simulink model "SIP_DynSys_Model_V1_0"  (R2024a)
settings: Solver=VariableStepAuto  StartTime=0.0  StopTime=10.0  RelTol=1e-3
settings Model: Creator=yunus  LastModifiedBy=yunus

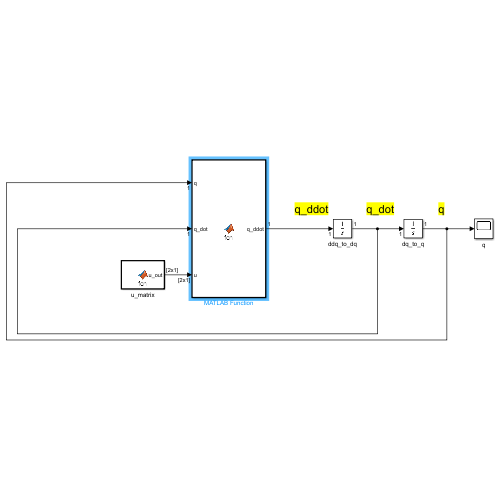
[thumbnail: Simulink's stored preview of the top-level diagram]
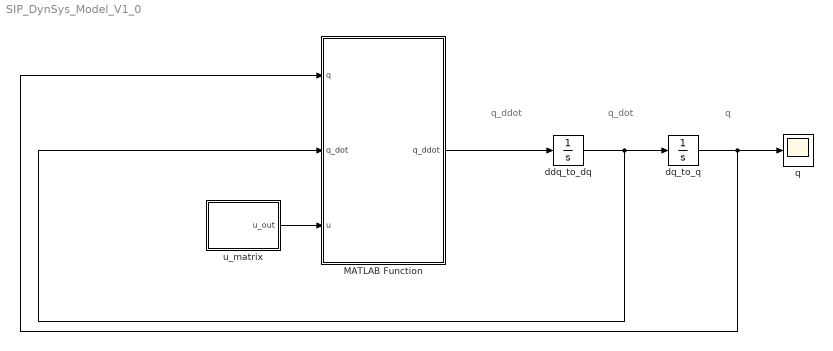
== system SIP_DynSys_Model_V1_0 ==
  note: q_ddot
  note: q
  note: q_dot
  MATLAB Function : MATLAB Function  TreatAsAtomicUnit=on
  ddq_to_dq : Integrator
  dq_to_q : Integrator  InitialCondition=0.4
  q : Scope
  u_matrix : MATLAB Function  TreatAsAtomicUnit=on
  wires:
  ddq_to_dq/1 -> MATLAB Function/2(q_dot), dq_to_q/1
  dq_to_q/1 -> MATLAB Function/1(q), q/1
  MATLAB Function/1(q_ddot) -> ddq_to_dq/1
  u_matrix/1(u_out) -> MATLAB Function/3(u)

== matlab function SIP_DynSys_Model_V1_0/u_matrix ==
  data: u_out output
function u_out = fcn()

u_out = [1;1];

== matlab function SIP_DynSys_Model_V1_0/MATLAB Function ==
  data: q input; q_ddot output; q_dot input; u input
function q_ddot = fcn(q, q_dot, u)
   
    % Predefine the size of q_ddot to avoid Simulink code generation errors.
    % Simulink requires the output size to be explicitly specified.
    q_ddot = zeros(8,1);

    % Calls the Dynamics function
    q_ddot = SIP_MotionSolver(q, q_dot, u);
    
end
